simulink model "c_FSF_LQR_Sim"  (R2018b)
settings: Solver=VariableStepAuto  StartTime=0.0  StopTime=10  RelTol=1e-3
values from neighbouring files (symbols this model uses):
  FSF_Inital = [0.1 0.2 0.01 0.5 0.6 0.2]    [d_Control_FSF_LQR_Design.m]
  K_FSF = place(A_Reform, B_Reform, Desired_Poles)    [d_Control_FSF_LQR_Design.m]
  K_LQR = lqr(A_Reform, B_Reform, Q, R)    [d_Control_FSF_LQR_Design.m]
  LQR_Inital = [0.1 0.2 0.01 0.5 0.6 0.2]    [d_Control_FSF_LQR_Design.m]
undefined symbols (not defined in the file or in its folder): A_Reform, B_Reform, C_Reform, D_Reform
settings Model: Creator=Milad  LastModifiedBy=Milad
settings DataIOCC: ReturnWorkspaceOutputs=on

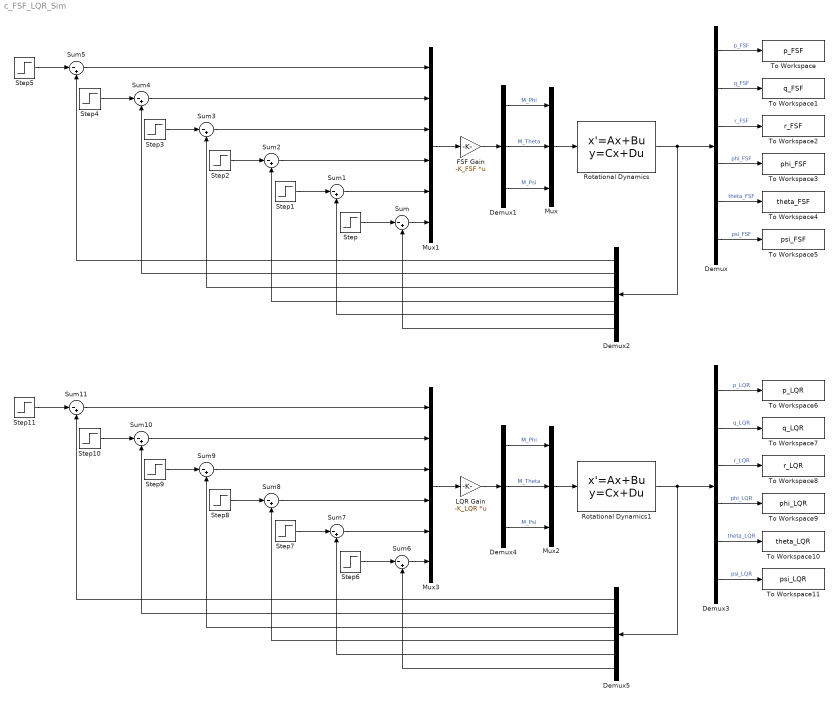
== system c_FSF_LQR_Sim ==
  Demux{,2..3,5} (4 alike) : Demux  Outputs=6
  Demux1 : Demux  Outputs=3
  Demux4 : Demux  Outputs=3
  FSF Gain : Gain  Gain=-K_FSF  Multiplication=Matrix(K*u)
  LQR Gain : Gain  Gain=-K_LQR  Multiplication=Matrix(K*u)
  Mux : Mux  Inputs=3
  Mux1 : Mux  Inputs=6
  Mux2 : Mux  Inputs=3
  Mux3 : Mux  Inputs=6
  Rotational Dynamics : StateSpace  A=A_Reform  B=B_Reform  C=C_Reform  D=D_Reform  InitialCondition=FSF_Inital
  Rotational Dynamics1 : StateSpace  A=A_Reform  B=B_Reform  C=C_Reform  D=D_Reform  InitialCondition=LQR_Inital
  Step : Step  Time=10  After=0  SampleTime=0
  Step{1..5,7..11} (10 alike) : Step  Time=0  After=0  SampleTime=0
  Step6 : Step  Time=10  After=0  SampleTime=0
  Sum{,1..11} (12 alike) : Sum  Inputs=|-+
  To Workspace : ToWorkspace  VariableName=p_FSF  SampleTime=-1
  To Workspace1 : ToWorkspace  VariableName=q_FSF  SampleTime=-1
  To Workspace10 : ToWorkspace  VariableName=theta_LQR  SampleTime=-1
  To Workspace11 : ToWorkspace  VariableName=psi_LQR  SampleTime=-1
  To Workspace2 : ToWorkspace  VariableName=r_FSF  SampleTime=-1
  To Workspace3 : ToWorkspace  VariableName=phi_FSF  SampleTime=-1
  To Workspace4 : ToWorkspace  VariableName=theta_FSF  SampleTime=-1
  To Workspace5 : ToWorkspace  VariableName=psi_FSF  SampleTime=-1
  To Workspace6 : ToWorkspace  VariableName=p_LQR  SampleTime=-1
  To Workspace7 : ToWorkspace  VariableName=q_LQR  SampleTime=-1
  To Workspace8 : ToWorkspace  VariableName=r_LQR  SampleTime=-1
  To Workspace9 : ToWorkspace  VariableName=phi_LQR  SampleTime=-1
  wires:
  FSF Gain/1 -> Demux1/1
  Mux1/1 -> FSF Gain/1
  Rotational Dynamics/1 -> Demux2/1, Demux/1
  Mux/1 -> Rotational Dynamics/1
  Demux1/1 -> Mux/1  "M_Phi"
  Demux1/2 -> Mux/2  "M_Theta"
  Demux1/3 -> Mux/3  "M_Psi"
  Demux/1 -> To Workspace/1  "p_FSF"
  Demux/2 -> To Workspace1/1  "q_FSF"
  Demux/3 -> To Workspace2/1  "r_FSF"
  Demux/4 -> To Workspace3/1  "phi_FSF"
  Demux/5 -> To Workspace4/1  "theta_FSF"
  Demux/6 -> To Workspace5/1  "psi_FSF"
  Step/1 -> Sum/1
  Sum/1 -> Mux1/6
  Sum1/1 -> Mux1/5
  Step1/1 -> Sum1/1
  Step2/1 -> Sum2/1
  Sum2/1 -> Mux1/4
  Sum3/1 -> Mux1/3
  Step3/1 -> Sum3/1
  Step4/1 -> Sum4/1
  Sum4/1 -> Mux1/2
  Sum5/1 -> Mux1/1
  Step5/1 -> Sum5/1
  Demux2/1 -> Sum5/2
  Demux2/2 -> Sum4/2
  Demux2/3 -> Sum3/2
  Demux2/4 -> Sum2/2
  Demux2/5 -> Sum1/2
  Demux2/6 -> Sum/2
  Demux5/6 -> Sum6/2
  Demux5/5 -> Sum7/2
  Demux5/4 -> Sum8/2
  Demux5/3 -> Sum9/2
  Demux5/2 -> Sum10/2
  Demux5/1 -> Sum11/2
  Step11/1 -> Sum11/1
  Sum11/1 -> Mux3/1
  Sum10/1 -> Mux3/2
  Step10/1 -> Sum10/1
  Step9/1 -> Sum9/1
  Sum9/1 -> Mux3/3
  Sum8/1 -> Mux3/4
  Step8/1 -> Sum8/1
  Step7/1 -> Sum7/1
  Sum7/1 -> Mux3/5
  Sum6/1 -> Mux3/6
  Step6/1 -> Sum6/1
  Demux3/6 -> To Workspace11/1  "psi_LQR"
  Demux3/5 -> To Workspace10/1  "theta_LQR"
  Demux3/4 -> To Workspace9/1  "phi_LQR"
  Demux3/3 -> To Workspace8/1  "r_LQR"
  Demux3/2 -> To Workspace7/1  "q_LQR"
  Demux3/1 -> To Workspace6/1  "p_LQR"
  Demux4/3 -> Mux2/3  "M_Psi"
  Demux4/2 -> Mux2/2  "M_Theta"
  Demux4/1 -> Mux2/1  "M_Phi"
  Mux2/1 -> Rotational Dynamics1/1
  Rotational Dynamics1/1 -> Demux3/1, Demux5/1
  Mux3/1 -> LQR Gain/1
  LQR Gain/1 -> Demux4/1
